simulink subsystem "Day1_Scenario_3_4"  (R2024a)
settings: Solver=VariableStepAuto  StartTime=0.0  StopTime=10.0  RelTol=1e-3
libraries: CarMaker4SL x3
settings Model: Creator=junhyung.cha  LastModifiedBy=User

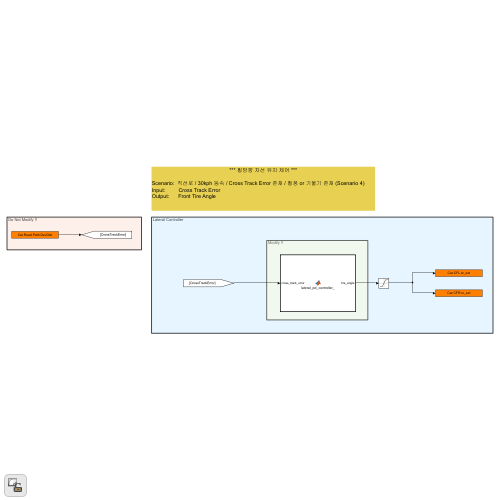
[thumbnail: Simulink's stored preview of the top-level diagram]
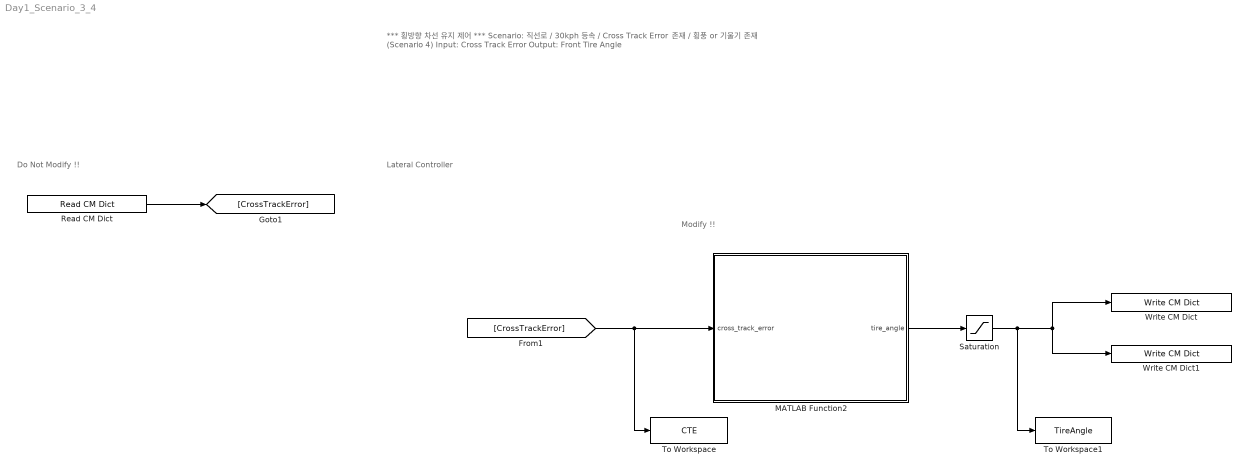
== system Day1_Scenario_3_4 ==
  note: Do Not Modify !!
  note: Modify !!
  note: Lateral Controller
  note: *** 횡방향 차선 유지 제어 ***
      |
      | Scenario: 직선로 / 30kph 등속 / Cross Track Error 존재 / 횡풍 or 기울기 존재 (Scenario 4)
      | Input: Cross Track Error
      | Output: Front Tire Angle
  MATLAB Function2 : MATLAB Function  TreatAsAtomicUnit=on
  Read CM Dict : CarMaker4SL/Read CM Dict  xname=Car.Road.Path.DevDist  xsync=off  xstime=Inherited
  Saturation : Saturate  UpperLimit=2  LowerLimit=-2
  To Workspace : ToWorkspace  VariableName=CTE  SaveFormat=Timeseries  SampleTime=-1
  To Workspace1 : ToWorkspace  VariableName=TireAngle  SaveFormat=Timeseries  SampleTime=-1
  Write CM Dict : CarMaker4SL/Write CM Dict  xname=Car.CFL.rz_ext  xsync=off
  Write CM Dict1 : CarMaker4SL/Write CM Dict  xname=Car.CFR.rz_ext  xsync=off
  wires:
  Read CM Dict/1 -> [CrossTrackError]
  MATLAB Function2/1(tire_angle) -> Saturation/1
  [CrossTrackError] -> MATLAB Function2/1(cross_track_error), To Workspace/1
  Saturation/1 -> Write CM Dict/1, Write CM Dict1/1, To Workspace1/1

== matlab function Day1_Scenario_3_4/MATLAB Function2 ==
  settings: updateMethod=DISCRETE  sampleTime=0.05
  data: cross_track_error input; tire_angle output
function tire_angle = lateral_pd_controller_(cross_track_error)
    tire_angle = lateral_pd_controller_mfile(cross_track_error);
end


function tire_angle = lateral_pd_controller_mfile(cross_track_error)
    persistent error_prev error_sum
    % error = average_filter_mfile(cross_track_error);
    error = cross_track_error;
    dt = 0.05;

    if isempty(error_prev)
        error_prev = error;
    end

    if isempty(error_sum)
        error_sum = 0;
    else
        error_sum = error_sum + error * dt;
    end

    Kp = 0.415;
    Ki = 0.001;
    Kd = 0.25;
    
    P_term = Kp*error;
    I_term = Ki*error_sum;
    D_term = Kd*(error - error_prev) / dt;
    
    tire_angle = -(P_term + I_term + D_term);
    error_prev = error;
end
